simulink model "dynamics"  (R2024a)
settings: Solver=VariableStepAuto  StartTime=0.0  StopTime=10.0  RelTol=1e-3
values from neighbouring files (symbols this model uses):
  Arm = [ ... (first row only)    [launch.m]
  CDDrone = 0.01    [launch.m]
  CDval = 0.008    [launch.m]
  g = 9.81    [launch.m]
  m = 1    [launch.m]
  prop_inertia = (1/12) * 0.015 * 0.127^2    (= 2.016125e-05)    [launch.m]
  R = 0.127    [launch.m]
  rotorRPMMax = 10000    [launch.m]
  rotorTimeConst = 0.05    [launch.m]
  SampleTime = 0.004    [launch.m]
  tilt_speed = [0; pi/4; 0]    [launch.m]
undefined symbols (not defined in the file or in its folder): contact, control, ddx, ddy, ddz, dx, dy, dz, lastVh, p, pitch, q, r, roll, X, Y, yaw, Z
libraries: simulink x2, shared6dof x1, simulink_extras x1, sharedutil x1, matrix_library x1
settings Model: Creator=tommy  LastModifiedBy=tommy

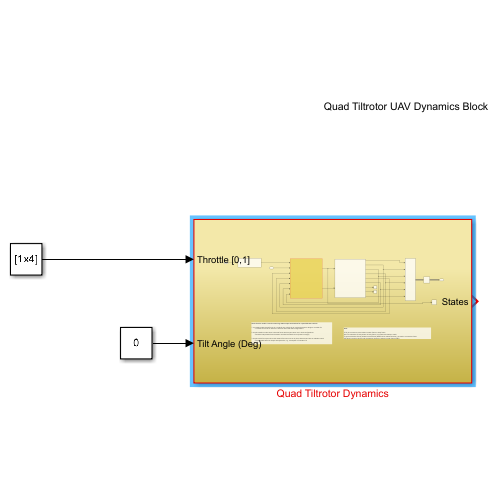
[thumbnail: Simulink's stored preview of the top-level diagram]
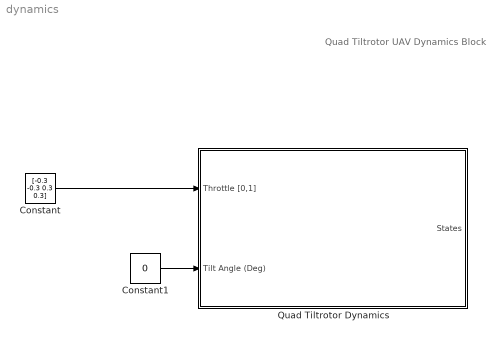
== system dynamics ==
  note: Quad Tiltrotor UAV Dynamics Block
  Constant : Constant  Value=[-0.3 -0.3 0.3 0.3]
  Constant1 : Constant  Value=0
  Quad Tiltrotor Dynamics : Subsystem
  wires:
  Constant/1 -> Quad Tiltrotor Dynamics/1(Throttle [0,1])
  Constant1/1 -> Quad Tiltrotor Dynamics/2(Tilt Angle (Deg))

== system dynamics/Quad Tiltrotor Dynamics ==
  note: Goals for this model : A novel vortex ring state escape mechanism for a quad tilt-rotor vehicle.
      |
      | 1. accurately portray thrust forces in a quad-tilt rotor vehicle in an in-place descent to design a controller for
      | - curve fits from CFD for descent in both non tilted and tilted configurations
      |
      | 2. simple transition model since horizontal forces and torques cancel out in both configurations
      | - transition interpolates forces between non tilted and tilted curves (based on angle)
      |
      | 3. simple model for torques since this research focuses more on in-place descents and less on attitude control
      | - torque model based on simple aerodynamics, e.g., assumption of constant Cd
  note: Note:
      |
      | DCM_be converts a vector written in earth frame to body frame
      | Abe is acceleration of body written in body frame, but measured relative to earth.
      | To get acceleration of body written in earth frame (NED fixed on takeoff location), we need to convert the frame.
      | IMU block's angular velocity and acceleration inputs are written in earth frame (NED)
  Throttle [0,1] : Inport
  Tilt Angle (Deg) : Inport  Port=2
  6DOF (Quaternion) : shared6dof/6DOF (Euler Angles)  units=Metric (MKS)  mtype=Fixed  rep=Quaternion  xme_0=init.posNED  Vm_0=init.vb  eul_0=init.euler  pm_0=init.angRates  mass_0=m  mass_e=0.5  mass_f=2.0  inertia=inertia  inertia_e=eye(3)  inertia_f=2*eye(3)  k_quat=1  vre_flag=on  abi_flag=on  aMode=0  xme_statename=''  Vm_statename=''  eul_statename=''  quat_statename=''  pm_statename=''  mass_statename=''
      settings: LibrarySourceBlock=aerolib6dof2/6DOF (Quaternion)
  Airframe : Subsystem
      mask Display: image('PX4-Quad-X-Motor-Configuration-33.png', [5,0,0,0,80,50]);
  Motor Model : Subsystem
  Rate Transition : RateTransition  OutPortSampleTime=SampleTime
  Scope : Scope
  States Bus : Subsystem
  Terminator : Terminator
  Terminator1 : Terminator
  States : Outport
  wires:
  States Bus/1(States) -> Rate Transition/1
  Rate Transition/1 -> States/1
  6DOF (Quaternion)/7 -> Terminator/1
  6DOF (Quaternion)/4 -> Airframe/4(DCMbe), States Bus/4(DCMbe)
  6DOF (Quaternion)/6 -> Airframe/6(Wb), States Bus/5(Wb)
  Airframe/1(F_cg) -> Scope/1, 6DOF (Quaternion)/1
  6DOF (Quaternion)/2 -> Airframe/5(Xe), States Bus/2(Xe)
  Airframe/2(M_cg) -> 6DOF (Quaternion)/2
  6DOF (Quaternion)/9 -> States Bus/6(acc_lnav)
  6DOF (Quaternion)/5 -> Airframe/3(Vb)
  6DOF (Quaternion)/8 -> Terminator1/1
  6DOF (Quaternion)/3 -> Airframe/7(rpy), States Bus/3(rpy)
  6DOF (Quaternion)/1 -> States Bus/1(Ve)
  Tilt Angle (Deg)/1 -> Airframe/2(Tilt Angle (Deg))
  Throttle [0,1]/1 -> Motor Model/1(Throttle)
  Motor Model/1(RPM) -> Airframe/1(rpm)

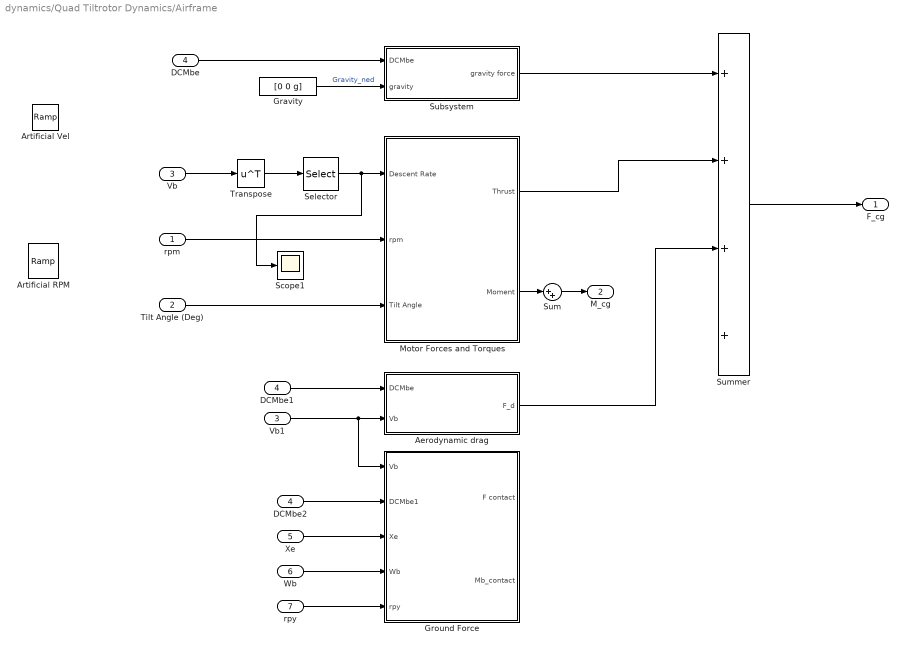
== system dynamics/Quad Tiltrotor Dynamics/Airframe ==
  rpm : Inport
  Tilt Angle (Deg) : Inport  Port=2
  Vb : Inport  Port=3
  DCMbe : Inport  Port=4
  Xe : Inport  Port=5
  Wb : Inport  Port=6
  rpy : Inport  Port=7
  Aerodynamic drag : Subsystem
  Artificial RPM : simulink/Sources/Ramp  slope=[0;-0;0;-0]  start=0  InitialOutput=[-3000; 3000; -2000; 2000]  VectorParams1D=off
  Artificial Vel : simulink/Sources/Ramp  slope=[0;0;0]  start=0  InitialOutput=[0;0;0]  VectorParams1D=off
  DCMbe1 : InportShadow  Port=4
  DCMbe2 : InportShadow  Port=4
  Gravity : Constant  Value=[0 0 g]
  Ground Force : Subsystem
  Motor Forces and Torques : Subsystem
  Scope1 : Scope
  Selector : Selector  InputPortWidth=3  IndexOptions=Index vector (dialog)  Indices=[3]  OutputSizes=1
  Subsystem : Subsystem
  Sum : Sum  Inputs=|++
  Summer : Sum  Inputs=++++
  Transpose : Math  Operator=transpose
  Vb1 : InportShadow  Port=3
  F_cg : Outport
  M_cg : Outport  Port=2
  wires:
  Subsystem/1(gravity force) -> Summer/1
  rpm/1 -> Motor Forces and Torques/2(rpm)
  Gravity/1 -> Subsystem/2(gravity)  "Gravity_ned"
  DCMbe/1 -> Subsystem/1(DCMbe)
  Transpose/1 -> Selector/1
  Selector/1 -> Scope1/1, Motor Forces and Torques/1(Descent Rate)
  Tilt Angle (Deg)/1 -> Motor Forces and Torques/3(Tilt Angle)
  Summer/1 -> F_cg/1
  Vb/1 -> Transpose/1
  DCMbe2/1 -> Ground Force/2(DCMbe1)
  Vb1/1 -> Ground Force/1(Vb), Aerodynamic drag/2(Vb)
  Xe/1 -> Ground Force/3(Xe)
  Aerodynamic drag/1(F_d) -> Summer/3
  Sum/1 -> M_cg/1
  rpy/1 -> Ground Force/5(rpy)
  Wb/1 -> Ground Force/4(Wb)
  DCMbe1/1 -> Aerodynamic drag/1(DCMbe)
  Motor Forces and Torques/2(Moment) -> Sum/1
  Motor Forces and Torques/1(Thrust) -> Summer/2

== system dynamics/Quad Tiltrotor Dynamics/Motor Model ==
  Throttle : Inport
  Demux : Demux
  Gain : Gain  Gain=[-1;-1;1;1]
  Mux : Mux
  Transfer Fcn{,2..4} (4 alike) : TransferFcn  Numerator=[rotorRPMMax]  Denominator=[rotorTimeConst 1]
  RPM : Outport
  wires:
  Mux/1 -> Gain/1
  Transfer Fcn/1 -> Mux/4
  Demux/4 -> Transfer Fcn/1
  Transfer Fcn3/1 -> Mux/2
  Transfer Fcn2/1 -> Mux/3
  Demux/1 -> Transfer Fcn4/1
  Demux/3 -> Transfer Fcn2/1
  Demux/2 -> Transfer Fcn3/1
  Transfer Fcn4/1 -> Mux/1
  Gain/1 -> RPM/1
  Throttle/1 -> Demux/1

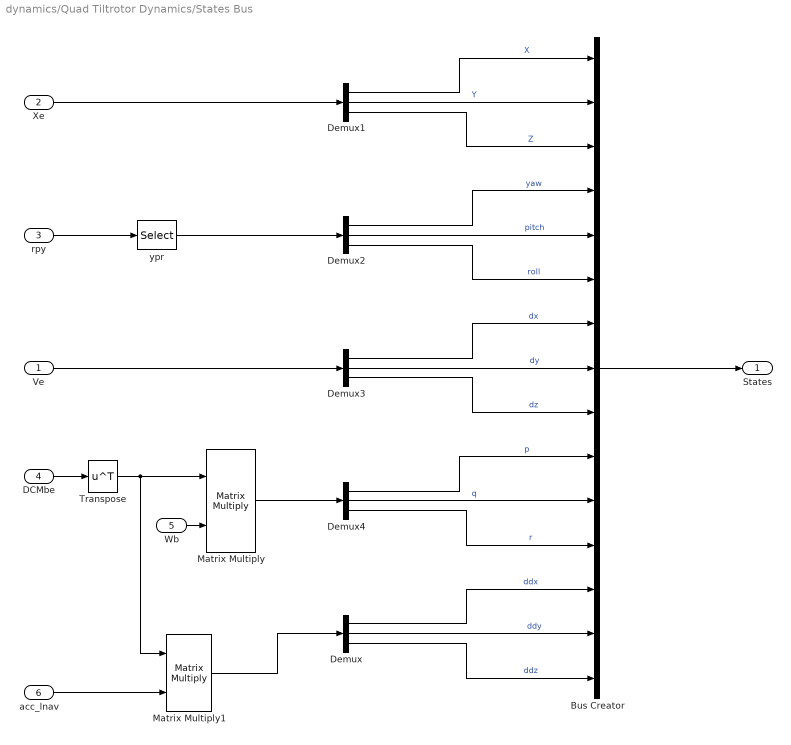
== system dynamics/Quad Tiltrotor Dynamics/States Bus ==
  Ve : Inport
  Xe : Inport  Port=2
  rpy : Inport  Port=3
  DCMbe : Inport  Port=4
  Wb : Inport  Port=5
  acc_lnav : Inport  Port=6
  Bus Creator : BusCreator  Inputs=X,Y,Z,yaw,pitch,roll,dx,dy,dz,p,q,r,ddx,ddy,ddz
  Demux{,1..4} (5 alike) : Demux  Outputs=3
  Matrix Multiply : Product  Multiplication=Matrix(*)
  Matrix Multiply1 : Product  Multiplication=Matrix(*)
  Transpose : Math  Operator=transpose
  ypr : Selector  InputPortWidth=3  IndexOptions=Index vector (dialog)  Indices=[3 2 1]  OutputSizes=1
  States : Outport
  wires:
  Demux1/1 -> Bus Creator/1  "X"
  Demux1/2 -> Bus Creator/2  "Y"
  rpy/1 -> ypr/1
  Demux2/2 -> Bus Creator/5  "pitch"
  Demux3/2 -> Bus Creator/8  "dy"
  Demux2/3 -> Bus Creator/6  "roll"
  Ve/1 -> Demux3/1
  Demux2/1 -> Bus Creator/4  "yaw"
  Demux1/3 -> Bus Creator/3  "Z"
  Demux3/1 -> Bus Creator/7  "dx"
  Demux4/2 -> Bus Creator/11  "q"
  Demux3/3 -> Bus Creator/9  "dz"
  Demux4/3 -> Bus Creator/12  "r"
  Demux4/1 -> Bus Creator/10  "p"
  Bus Creator/1 -> States/1
  Xe/1 -> Demux1/1
  Demux/3 -> Bus Creator/15  "ddz"
  Demux/2 -> Bus Creator/14  "ddy"
  Demux/1 -> Bus Creator/13  "ddx"
  Matrix Multiply/1 -> Demux4/1
  DCMbe/1 -> Transpose/1
  Transpose/1 -> Matrix Multiply1/1, Matrix Multiply/1
  Wb/1 -> Matrix Multiply/2
  acc_lnav/1 -> Matrix Multiply1/2
  Matrix Multiply1/1 -> Demux/1
  ypr/1 -> Demux2/1

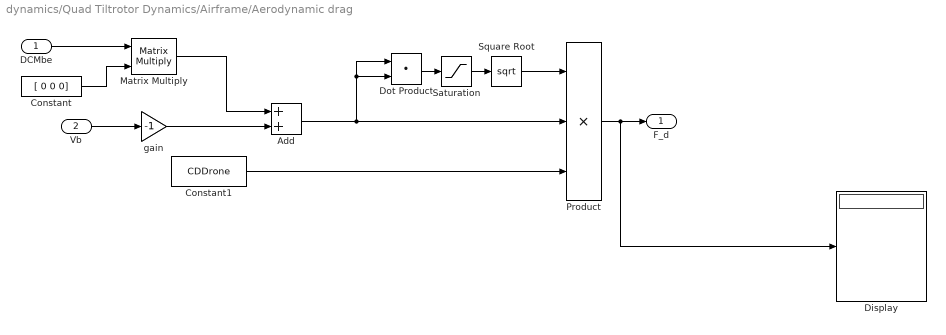
== system dynamics/Quad Tiltrotor Dynamics/Airframe/Aerodynamic drag ==
  DCMbe : Inport
  Vb : Inport  Port=2
  Add : Sum
  Constant : Constant  Value=[ 0 0 0]
  Constant1 : Constant  Value=CDDrone
  Display : Display
  Dot Product : DotProduct  OutDataTypeStr=Inherit: Inherit via internal rule
  Matrix Multiply : Product  Multiplication=Matrix(*)
  Product : Product  Inputs=3
  Saturation : Saturate  UpperLimit=inf  LowerLimit=0.0001
  Square Root : Sqrt
  gain : Gain  Gain=-1
  F_d : Outport
  wires:
  Saturation/1 -> Square Root/1
  Vb/1 -> gain/1
  Dot Product/1 -> Saturation/1
  Square Root/1 -> Product/1
  Constant1/1 -> Product/3
  DCMbe/1 -> Matrix Multiply/1
  Constant/1 -> Matrix Multiply/2
  gain/1 -> Add/2
  Matrix Multiply/1 -> Add/1
  Add/1 -> Dot Product/1, Dot Product/2, Product/2
  Product/1 -> Display/1, F_d/1

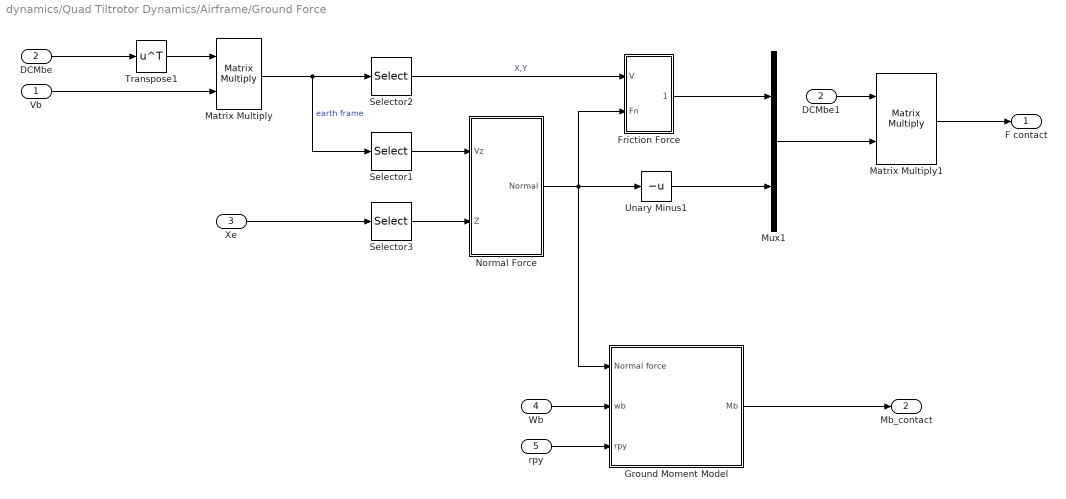
== system dynamics/Quad Tiltrotor Dynamics/Airframe/Ground Force ==
  Vb : Inport
  DCMbe1 : Inport  Port=2
  Xe : Inport  Port=3
  Wb : Inport  Port=4
  rpy : Inport  Port=5
  DCMbe : InportShadow  Port=2
  Friction Force : Subsystem
  Ground Moment Model : Subsystem
  Matrix Multiply : Product  Multiplication=Matrix(*)
  Matrix Multiply1 : Product  Multiplication=Matrix(*)
  Mux1 : Mux  Inputs=2
  Normal Force : Subsystem
  Selector1 : Selector  InputPortWidth=3  IndexOptions=Index vector (dialog)  Indices=[3]  OutputSizes=1
  Selector2 : Selector  InputPortWidth=3  IndexOptions=Index vector (dialog)  Indices=[1,2]  OutputSizes=1
  Selector3 : Selector  InputPortWidth=3  IndexOptions=Index vector (dialog)  Indices=[3]  OutputSizes=1
  Transpose1 : Math  Operator=transpose
  Unary Minus1 : UnaryMinus
  F contact : Outport
  Mb_contact : Outport  Port=2
  wires:
  Matrix Multiply1/1 -> F contact/1
  Friction Force/1(Friction) -> Mux1/1
  Xe/1 -> Selector3/1
  Vb/1 -> Matrix Multiply/2
  Selector3/1 -> Normal Force/2(Z)
  Matrix Multiply/1 -> Selector1/1, Selector2/1  "earth frame"
  Mux1/1 -> Matrix Multiply1/2
  Selector2/1 -> Friction Force/1(V)  "X,Y"
  Selector1/1 -> Normal Force/1(Vz)
  DCMbe1/1 -> Matrix Multiply1/1
  DCMbe/1 -> Transpose1/1
  Transpose1/1 -> Matrix Multiply/1
  Unary Minus1/1 -> Mux1/2
  Normal Force/1(Normal) -> Ground Moment Model/1(Normal force), Unary Minus1/1, Friction Force/2(Fn)
  Wb/1 -> Ground Moment Model/2(wb)
  rpy/1 -> Ground Moment Model/3(rpy)
  Ground Moment Model/1(Mb) -> Mb_contact/1

== system dynamics/Quad Tiltrotor Dynamics/Airframe/Motor Forces and Torques ==
  Descent Rate : Inport
  rpm : Inport  Port=2
  Tilt Angle : Inport  Port=3
  Constant1 : Constant  Value=Arm
  Degrees to Radians : simulink_extras/Transformations/Degrees to Radians
  Multirotor Subsystem : Subsystem  TreatAsAtomicUnit=on
  Sum of Elements : Sum  Inputs=+  CollapseMode=Specified dimension  CollapseDim=2
  Sum of Elements1 : Sum  Inputs=+  CollapseMode=Specified dimension  CollapseDim=2
  rho : Constant  Value=1.225
  Thrust : Outport
  Moment : Outport  Port=2
  wires:
  Tilt Angle/1 -> Degrees to Radians/1
  Constant1/1 -> Multirotor Subsystem/4(Arm)
  Degrees to Radians/1 -> Multirotor Subsystem/5(Tilt Angle (rad))
  Sum of Elements/1 -> Thrust/1
  Sum of Elements1/1 -> Moment/1
  Descent Rate/1 -> Multirotor Subsystem/1(Descent Rate (+ve down))
  rho/1 -> Multirotor Subsystem/2(rho)
  Multirotor Subsystem/2(Moment) -> Sum of Elements1/1
  Multirotor Subsystem/1(Thrust) -> Sum of Elements/1
  rpm/1 -> Multirotor Subsystem/3(rpm)

== system dynamics/Quad Tiltrotor Dynamics/Airframe/Subsystem ==
  DCMbe : Inport
  gravity : Inport  Port=2  Unit=m/s^2
  Gain1 : Gain  Gain=m
  Product : Product  Multiplication=Matrix(*)
  gravity force : Outport  Unit=N  VectorParamsAs1DForOutWhenUnconnected=off
  wires:
  gravity/1 -> Gain1/1
  Product/1 -> gravity force/1
  DCMbe/1 -> Product/1
  Gain1/1 -> Product/2  "gravity force NED"

== system dynamics/Quad Tiltrotor Dynamics/Airframe/Ground Force/Friction Force ==
  V : Inport
  Fn : Inport  Port=2
  Product : Product
  Saturation : Saturate  UpperLimit=contact.translation.maxFriction  LowerLimit=-contact.translation.maxFriction
  Soft Coulomb Friction : Subsystem
  Unary Minus : UnaryMinus
  Friction : Outport
  wires:
  Fn/1 -> Product/2
  Soft Coulomb Friction/1(Out1) -> Product/1
  Product/1 -> Unary Minus/1
  V/1 -> Soft Coulomb Friction/1(In1)
  Unary Minus/1 -> Saturation/1
  Saturation/1 -> Friction/1

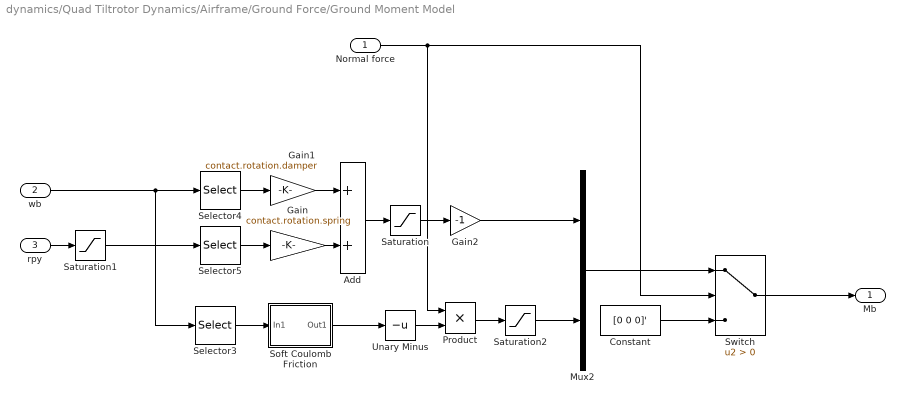
== system dynamics/Quad Tiltrotor Dynamics/Airframe/Ground Force/Ground Moment Model ==
  Normal force : Inport
  wb : Inport  Port=2
  rpy : Inport  Port=3
  Add : Sum
  Constant : Constant  Value=[0 0 0]'
  Gain : Gain  Gain=contact.rotation.spring
  Gain1 : Gain  Gain=contact.rotation.damper
  Gain2 : Gain  Gain=-1
  Mux2 : Mux  Inputs=2
  Product : Product
  Saturation : Saturate  UpperLimit=control.rotation.maxMoment  LowerLimit=-control.rotation.maxMoment
  Saturation1 : Saturate  UpperLimit=20*pi/180  LowerLimit=-20*pi/180
  Saturation2 : Saturate  UpperLimit=control.rotation.maxMoment  LowerLimit=-control.rotation.maxMoment
  Selector3 : Selector  InputPortWidth=3  IndexOptions=Index vector (dialog)  Indices=[3]  OutputSizes=1
  Selector4 : Selector  InputPortWidth=3  IndexOptions=Index vector (dialog)  Indices=[1, 2]  OutputSizes=1
  Selector5 : Selector  InputPortWidth=3  IndexOptions=Index vector (dialog)  Indices=[1, 2]  OutputSizes=1
  Soft Coulomb Friction : Subsystem
  Switch : Switch  Criteria=u2 > Threshold  SaturateOnIntegerOverflow=off  InputSameDT=off
  Unary Minus : UnaryMinus
  Mb : Outport
  wires:
  Gain2/1 -> Mux2/1
  Add/1 -> Saturation/1
  Gain/1 -> Add/2
  Saturation/1 -> Gain2/1
  Selector4/1 -> Gain1/1
  Gain1/1 -> Add/1
  Constant/1 -> Switch/3
  Selector5/1 -> Gain/1
  Switch/1 -> Mb/1
  Mux2/1 -> Switch/1
  Normal force/1 -> Product/1, Switch/2
  rpy/1 -> Saturation1/1
  Saturation1/1 -> Selector5/1
  wb/1 -> Selector4/1, Selector3/1
  Selector3/1 -> Soft Coulomb Friction/1(In1)
  Soft Coulomb Friction/1(Out1) -> Unary Minus/1
  Unary Minus/1 -> Product/2
  Product/1 -> Saturation2/1
  Saturation2/1 -> Mux2/2

== system dynamics/Quad Tiltrotor Dynamics/Airframe/Ground Force/Normal Force ==
  Vz : Inport
  Z : Inport  Port=2
  Add : Sum
  Constant : Constant  Value=0
  Damper Kp : Gain  Gain=-contact.translation.damper
  Saturation : Saturate  UpperLimit=contact.translation.maxNormal  LowerLimit=0
  Spring Kp : Gain  Gain=-contact.translation.spring
  Switch : Switch  Criteria=u2 > Threshold  SaturateOnIntegerOverflow=off  InputSameDT=off
  Unary Minus : UnaryMinus
  Unary Minus1 : UnaryMinus
  Normal : Outport
  wires:
  Constant/1 -> Switch/1
  Z/1 -> Unary Minus/1
  Switch/1 -> Saturation/1
  Damper Kp/1 -> Add/2
  Add/1 -> Switch/3
  Spring Kp/1 -> Add/1
  Vz/1 -> Unary Minus1/1
  Saturation/1 -> Normal/1
  Unary Minus/1 -> Spring Kp/1, Switch/2
  Unary Minus1/1 -> Damper Kp/1

== system dynamics/Quad Tiltrotor Dynamics/Airframe/Motor Forces and Torques/Multirotor Subsystem ==
  Descent Rate (+ve down) : Inport
  rho : Inport  Port=2
  rpm : Inport  Port=3  Partition=on  PartitionDimension=1  PartitionWidth=1  PartitionOffset=0
  Arm : Inport  Port=4  Partition=on  PartitionDimension=2  PartitionWidth=1  PartitionOffset=0
  Tilt Angle (rad) : Inport  Port=5
  For Each : ForEach  DisableCoverage=on
  Rotor Subsystem : Subsystem
  Thrust : Outport  ConcatenationDimension=2
  Moment : Outport  Port=2  ConcatenationDimension=2
  wires:
  Rotor Subsystem/4(Mxyz) -> Moment/1  "Moment"
  Arm/1 -> Rotor Subsystem/4(Arm)
  Descent Rate (+ve down)/1 -> Rotor Subsystem/1(Descent Rate (+ve down))
  rho/1 -> Rotor Subsystem/2(rho)
  Rotor Subsystem/3(Fxyz) -> Thrust/1  "Thrust"
  rpm/1 -> Rotor Subsystem/3(rpm)
  Tilt Angle (rad)/1 -> Rotor Subsystem/5(Tilt Angle (rad))

== system dynamics/Quad Tiltrotor Dynamics/Airframe/Ground Force/Friction Force/Soft Coulomb Friction ==
  note: Pennestrì, E., Rossi, V., Salvini, P. et al. Review and comparison of dry friction force models. Nonlinear Dyn 83, 1785–1801 (2016). https://doi.org/10.1007/s11071-015-2485-3
  In1 : Inport
  Tanh : Trigonometry  Operator=tanh
  friction coefficient : Gain  Gain=contact.translation.friction
  vd : Gain  Gain=1/contact.translation.vd
  Out1 : Outport
  wires:
  In1/1 -> vd/1
  vd/1 -> Tanh/1
  Tanh/1 -> friction coefficient/1
  friction coefficient/1 -> Out1/1

== system dynamics/Quad Tiltrotor Dynamics/Airframe/Ground Force/Ground Moment Model/Soft Coulomb Friction ==
  note: Pennestrì, E., Rossi, V., Salvini, P. et al. Review and comparison of dry friction force models. Nonlinear Dyn 83, 1785–1801 (2016). https://doi.org/10.1007/s11071-015-2485-3
  In1 : Inport
  Tanh : Trigonometry  Operator=tanh
  friction coefficient : Gain  Gain=control.rotation.friction
  vd : Gain  Gain=1/control.rotation.vd
  Out1 : Outport
  wires:
  In1/1 -> vd/1
  vd/1 -> Tanh/1
  Tanh/1 -> friction coefficient/1
  friction coefficient/1 -> Out1/1

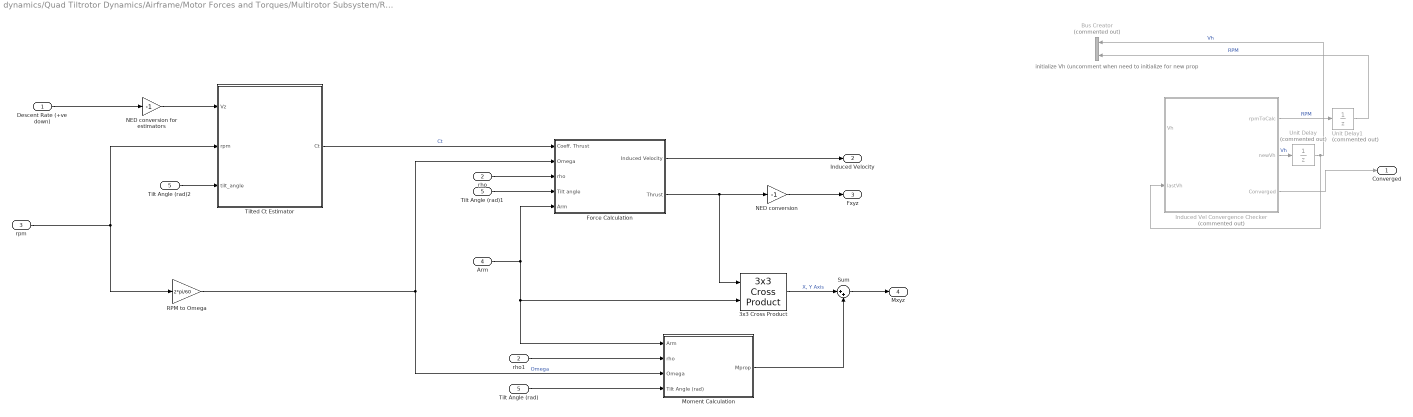
== system dynamics/Quad Tiltrotor Dynamics/Airframe/Motor Forces and Torques/Multirotor Subsystem/Rotor Subsystem ==
  note: initialize Vh (uncomment when need to initialize for new prop
  Descent Rate (+ve down) : Inport
  rho : Inport  Port=2
  rpm : Inport  Port=3
  Arm : Inport  Port=4
  Tilt Angle (rad) : Inport  Port=5
  3x3 Cross Product : sharedutil/3x3 Cross Product  aMode=aMode
      settings: LibrarySourceBlock=aerolibutil/3x3 Cross Product
  Bus Creator : BusCreator  Commented=on  Inputs=2
  Force Calculation : Subsystem
  Induced Vel Convergence Checker : MATLAB Function  Commented=on  TreatAsAtomicUnit=on  mask{VhInit=4.7, ConvThresh=1e-4}
      mask prompts: VhInit "Initial Vh Guess"; ConvThresh "Convergence Threshold"
  Moment Calculation : Subsystem
  NED conversion : Gain  Gain=-1
  NED conversion for estimators : Gain  Gain=-1
  RPM to Omega : Gain  Gain=2*pi/60
  Sum : Sum  Inputs=|++
  Tilt Angle (rad)1 : InportShadow  Port=5
  Tilt Angle (rad)2 : InportShadow  Port=5
  Tilted Ct Estimator : Subsystem
  Unit Delay : UnitDelay  Commented=on  InitialCondition=lastVh  SampleTime=0.001  HasFrameUpgradeWarning=on
  Unit Delay1 : UnitDelay  Commented=on  InitialCondition=1  SampleTime=0.001  HasFrameUpgradeWarning=on
  rho1 : InportShadow  Port=2
  Converged : Outport
  Induced Velocity : Outport  Port=2
  Fxyz : Outport  Port=3
  Mxyz : Outport  Port=4
  wires:
  Tilted Ct Estimator/1(Ct) -> Force Calculation/1(Coeff. Thrust)  "Ct"
  Unit Delay/1 -> Bus Creator/1, Induced Vel Convergence Checker/2(lastVh)  "Vh"
  Induced Vel Convergence Checker/3(Converged) -> Converged/1
  RPM to Omega/1 -> Moment Calculation/3(Omega), Force Calculation/2(Omega)  "Omega"
  rho/1 -> Force Calculation/3(rho)
  Induced Vel Convergence Checker/2(newVh) -> Unit Delay/1  "Vh"
  rpm/1 -> RPM to Omega/1, Tilted Ct Estimator/2(rpm)
  Descent Rate (+ve down)/1 -> NED conversion for estimators/1
  Unit Delay1/1 -> Bus Creator/2  "RPM"
  Induced Vel Convergence Checker/1(rpmToCalc) -> Unit Delay1/1  "RPM"
  Force Calculation/1(Induced Velocity) -> Induced Velocity/1
  Force Calculation/2(Thrust) -> NED conversion/1, 3x3 Cross Product/1
  3x3 Cross Product/1 -> Sum/1  "X, Y Axis"
  rho1/1 -> Moment Calculation/2(rho)
  Arm/1 -> 3x3 Cross Product/2, Moment Calculation/1(Arm), Force Calculation/5(Arm)
  Moment Calculation/1(Mprop) -> Sum/2
  Sum/1 -> Mxyz/1
  NED conversion/1 -> Fxyz/1
  Tilt Angle (rad)/1 -> Moment Calculation/4(Tilt Angle (rad))
  Tilt Angle (rad)1/1 -> Force Calculation/4(Tilt angle)
  NED conversion for estimators/1 -> Tilted Ct Estimator/1(Vz)
  Tilt Angle (rad)2/1 -> Tilted Ct Estimator/3(tilt_angle)

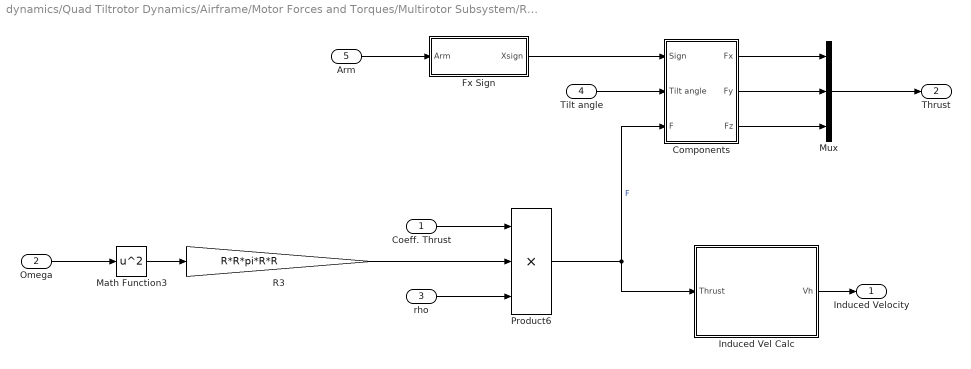
== system dynamics/Quad Tiltrotor Dynamics/Airframe/Motor Forces and Torques/Multirotor Subsystem/Rotor Subsystem/Force Calculation ==
  Coeff. Thrust : Inport
  Omega : Inport  Port=2
  rho : Inport  Port=3
  Tilt angle : Inport  Port=4
  Arm : Inport  Port=5
  Components : Subsystem
  Fx Sign : Subsystem
  Induced Vel Calc : Subsystem
  Math Function3 : Math  Operator=square  SignedPower=on
  Mux : Mux  Inputs=3
  Product6 : Product  Inputs=3
  R3 : Gain  Gain=R*R*pi*R*R
  Induced Velocity : Outport
  Thrust : Outport  Port=2
  wires:
  Coeff. Thrust/1 -> Product6/1
  Math Function3/1 -> R3/1
  Induced Vel Calc/1(Vh) -> Induced Velocity/1
  R3/1 -> Product6/2
  rho/1 -> Product6/3
  Omega/1 -> Math Function3/1
  Product6/1 -> Components/3(F), Induced Vel Calc/1(Thrust)  "F"
  Arm/1 -> Fx Sign/1(Arm)
  Mux/1 -> Thrust/1
  Fx Sign/1(Xsign) -> Components/1(Sign)
  Tilt angle/1 -> Components/2(Tilt angle)
  Components/1(Fx) -> Mux/1
  Components/2(Fy) -> Mux/2
  Components/3(Fz) -> Mux/3

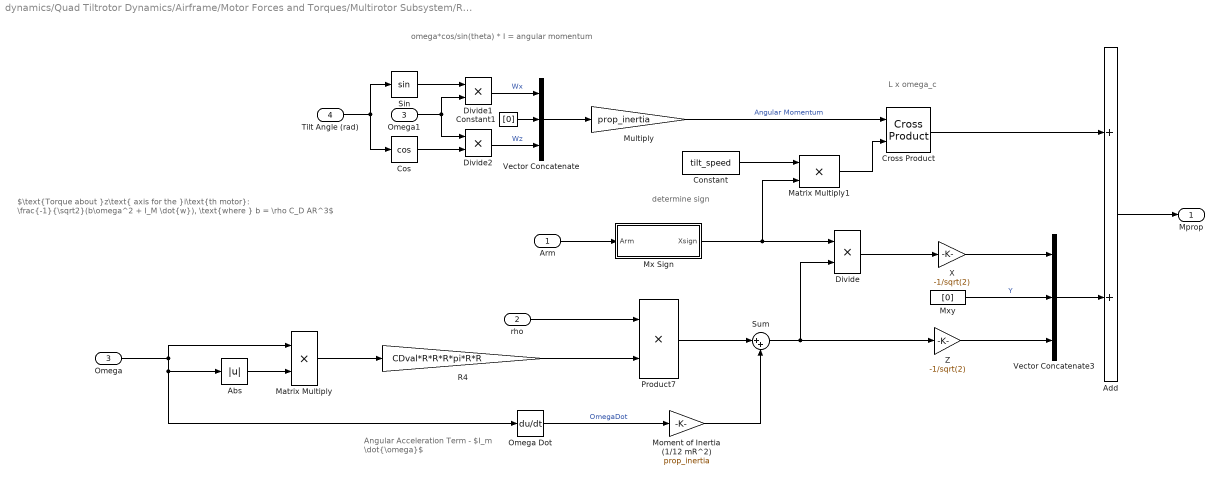
== system dynamics/Quad Tiltrotor Dynamics/Airframe/Motor Forces and Torques/Multirotor Subsystem/Rotor Subsystem/Moment Calculation ==
  note: determine sign
  note: L x omega_c
  note: omega*cos/sin(theta) * I = angular momentum
  note: $\text{Torque about }z\text{ axis for the }i\text{th motor}: \frac{-1}{\sqrt2}(b\omega^2 + I_M \dot{w}), \text{where } b = \rho C_D AR^3$
  note: Angular Acceleration Term - $I_m \dot{\omega}$
  Arm : Inport
  rho : Inport  Port=2
  Omega : Inport  Port=3
  Tilt Angle (rad) : Inport  Port=4
  Abs : Abs  SaturateOnIntegerOverflow=off
  Add : Sum
  Constant : Constant  Value=tilt_speed
  Constant1 : Constant  Value=[0]
  Cos : Trigonometry  Operator=cos
  Cross Product : matrix_library/Cross Product
  Divide : Product  Inputs=**
  Divide1 : Product  Inputs=**
  Divide2 : Product  Inputs=**
  Matrix Multiply : Product
  Matrix Multiply1 : Product
  Moment of Inertia (1/12 mR^2) : Gain  Gain=prop_inertia
  Multiply : Gain  Gain=prop_inertia
  Mx Sign : Subsystem
  Mxy : Constant  Value=[0]
  Omega Dot : Derivative
  Omega1 : InportShadow  Port=3
  Product7 : Product
  R4 : Gain  Gain=CDval*R*R*R*pi*R*R
  Sin : Trigonometry
  Sum : Sum  Inputs=|++
  Vector Concatenate : Concatenate  NumInputs=3
  Vector Concatenate3 : Concatenate  NumInputs=3
  X : Gain  Gain=-1/sqrt(2)
  Z : Gain  Gain=-1/sqrt(2)
  Mprop : Outport
  wires:
  R4/1 -> Product7/2
  rho/1 -> Product7/1
  Omega/1 -> Omega Dot/1, Abs/1, Matrix Multiply/1
  Omega Dot/1 -> Moment of Inertia (1/12 mR^2)/1  "OmegaDot"
  Sum/1 -> Z/1, Divide/2
  Product7/1 -> Sum/1
  Moment of Inertia (1/12 mR^2)/1 -> Sum/2
  Z/1 -> Vector Concatenate3/3
  Divide/1 -> X/1
  Mxy/1 -> Vector Concatenate3/2  "Y"
  Arm/1 -> Mx Sign/1(Arm)
  Mx Sign/1(Xsign) -> Divide/1, Matrix Multiply1/2
  Matrix Multiply/1 -> R4/1
  Abs/1 -> Matrix Multiply/2
  Tilt Angle (rad)/1 -> Cos/1, Sin/1
  Cos/1 -> Divide2/2
  Sin/1 -> Divide1/1
  Divide1/1 -> Vector Concatenate/1  "Wx"
  Vector Concatenate/1 -> Multiply/1
  Multiply/1 -> Cross Product/1  "Angular Momentum"
  Cross Product/1 -> Add/1
  Divide2/1 -> Vector Concatenate/3  "Wz"
  Constant1/1 -> Vector Concatenate/2
  Omega1/1 -> Divide2/1, Divide1/2
  Matrix Multiply1/1 -> Cross Product/2
  Constant/1 -> Matrix Multiply1/1
  X/1 -> Vector Concatenate3/1
  Vector Concatenate3/1 -> Add/2
  Add/1 -> Mprop/1

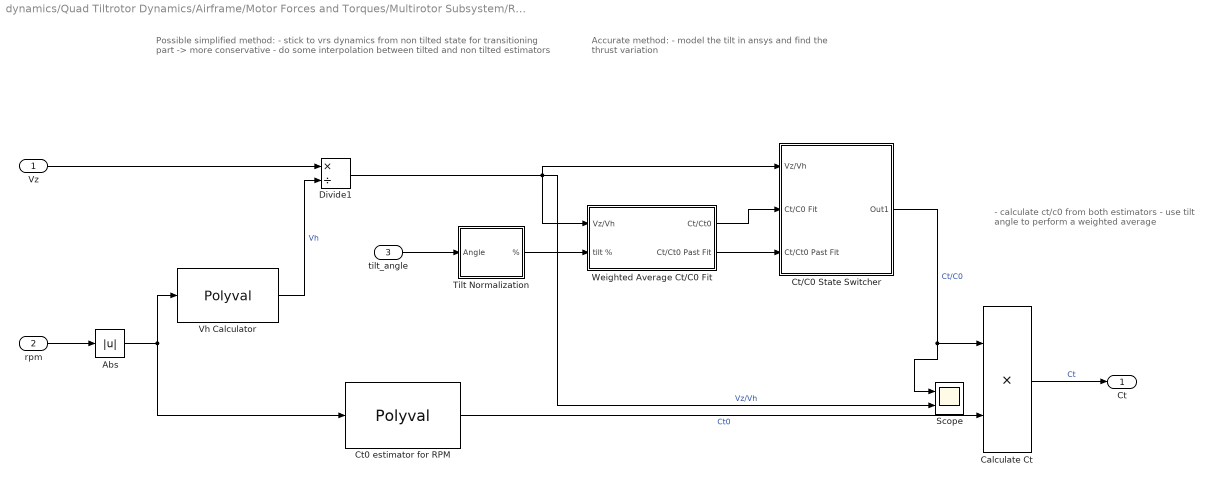
== system dynamics/Quad Tiltrotor Dynamics/Airframe/Motor Forces and Torques/Multirotor Subsystem/Rotor Subsystem/Tilted Ct Estimator ==
  note: - calculate ct/c0 from both estimators
      | - use tilt angle to perform a weighted average
  note: Accurate method:
      |
      | - model the tilt in ansys and find the thrust variation
  note: Possible simplified method:
      |
      | - stick to vrs dynamics from non tilted state for transitioning part -> more conservative
      | - do some interpolation between tilted and non tilted estimators
  Vz : Inport
  rpm : Inport  Port=2
  tilt_angle : Inport  Port=3
  Abs : Abs  SaturateOnIntegerOverflow=off
  Calculate Ct : Product  Inputs=**
  Ct/C0 State Switcher : Subsystem
  Ct0 estimator for RPM : Polyval  Coefs=[0.000000000012185, -0.000000274732884, 0.008305365728125]
  Divide1 : Product  Inputs=*/
  Scope : Scope  NumInputPorts=2
  Tilt Normalization : Subsystem
  Vh Calculator : Polyval  Coefs=[-5.17622414362771e-09, 0.000822973507549008, 0.0232660553338375]
  Weighted Average Ct/C0 Fit : Subsystem
  Ct : Outport
  wires:
  Vh Calculator/1 -> Divide1/2  "Vh"
  Ct/C0 State Switcher/1(Out1) -> Scope/1, Calculate Ct/1  "Ct/C0"
  Divide1/1 -> Scope/2, Ct/C0 State Switcher/1(" Vz/Vh"), Weighted Average Ct/C0 Fit/1(Vz/Vh)  "Vz/Vh"
  rpm/1 -> Abs/1
  Abs/1 -> Vh Calculator/1, Ct0 estimator for RPM/1
  Ct0 estimator for RPM/1 -> Calculate Ct/2  "Ct0"
  Vz/1 -> Divide1/1
  Calculate Ct/1 -> Ct/1  "Ct"
  Weighted Average Ct/C0 Fit/1(Ct/Ct0) -> Ct/C0 State Switcher/2(Ct/C0 Fit)
  tilt_angle/1 -> Tilt Normalization/1(Angle)
  Tilt Normalization/1(%) -> Weighted Average Ct/C0 Fit/2(tilt %)
  Weighted Average Ct/C0 Fit/2(Ct/Ct0 Past Fit) -> Ct/C0 State Switcher/3(Ct/Ct0 Past Fit)

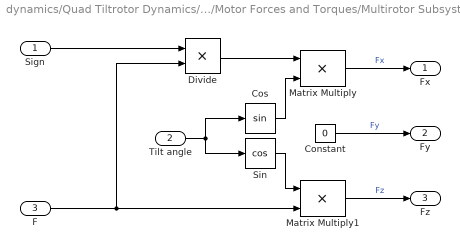
== system dynamics/Quad Tiltrotor Dynamics/Airframe/Motor Forces and Torques/Multirotor Subsystem/Rotor Subsystem/Force Calculation/Components ==
  Sign : Inport
  Tilt angle : Inport  Port=2
  F : Inport  Port=3
  Constant : Constant  Value=0
  Cos : Trigonometry
  Divide : Product  Inputs=**
  Matrix Multiply : Product
  Matrix Multiply1 : Product
  Sin : Trigonometry  Operator=cos
  Fx : Outport
  Fy : Outport  Port=2
  Fz : Outport  Port=3
  wires:
  Tilt angle/1 -> Cos/1, Sin/1
  Sign/1 -> Divide/1
  Sin/1 -> Matrix Multiply1/1
  Constant/1 -> Fy/1  "Fy"
  Cos/1 -> Matrix Multiply/2
  Matrix Multiply/1 -> Fx/1  "Fx"
  Divide/1 -> Matrix Multiply/1
  F/1 -> Matrix Multiply1/2, Divide/2
  Matrix Multiply1/1 -> Fz/1  "Fz"

== system dynamics/Quad Tiltrotor Dynamics/Airframe/Motor Forces and Torques/Multirotor Subsystem/Rotor Subsystem/Force Calculation/Fx Sign ==
  Arm : Inport
  Sign : Signum
  X selector : Selector  InputPortWidth=3  IndexOptions=Index vector (dialog)  Indices=[1]  OutputSizes=1
  Xsign : Outport
  wires:
  Arm/1 -> X selector/1
  X selector/1 -> Sign/1
  Sign/1 -> Xsign/1

== system dynamics/Quad Tiltrotor Dynamics/Airframe/Motor Forces and Torques/Multirotor Subsystem/Rotor Subsystem/Force Calculation/Induced Vel Calc ==
  Thrust : Inport
  Denom : Constant  Value=2*1.225*pi*R^2
  Divide : Product  Inputs=*/
  Saturation : Saturate  UpperLimit=inf  LowerLimit=0.0001
  Sqrt : Sqrt  OutDataTypeStr=double
  Vh : Outport
  wires:
  Denom/1 -> Divide/2
  Divide/1 -> Saturation/1
  Sqrt/1 -> Vh/1
  Thrust/1 -> Divide/1
  Saturation/1 -> Sqrt/1

== system dynamics/Quad Tiltrotor Dynamics/Airframe/Motor Forces and Torques/Multirotor Subsystem/Rotor Subsystem/Moment Calculation/Mx Sign ==
  Arm : Inport
  Sign : Signum
  X selector : Selector  InputPortWidth=3  IndexOptions=Index vector (dialog)  Indices=[1]  OutputSizes=1
  Xsign : Outport
  wires:
  Arm/1 -> X selector/1
  X selector/1 -> Sign/1
  Sign/1 -> Xsign/1

== system dynamics/Quad Tiltrotor Dynamics/Airframe/Motor Forces and Torques/Multirotor Subsystem/Rotor Subsystem/Tilted Ct Estimator/Ct//C0 State Switcher ==
  " Vz/Vh" : Inport
  Ct/C0 Fit : Inport  Port=2
  Ct/Ct0 Past Fit : Inport  Port=3
  Constant : Constant  Value=1.00463796511
  If : If  IfExpression=u1 >= -2 & u1 <= 0  ElseIfExpressions=u1 < -2
  If Action Subsystem : Subsystem  TreatAsAtomicUnit=on
  If Action Subsystem1 : Subsystem  TreatAsAtomicUnit=on
  If Action Subsystem2 : Subsystem  TreatAsAtomicUnit=on
  Merge : Merge  Inputs=3
  Out1 : Outport
  wires:
  If Action Subsystem1/1(" ") -> Merge/2
  If Action Subsystem2/1(Out1) -> Merge/3
  If/3 -> If Action Subsystem2/Action  "climb"
  If/1 -> If Action Subsystem/Action  "descent"
  If Action Subsystem/1(Out1) -> Merge/1
  " Vz/Vh"/1 -> If/1
  If/2 -> If Action Subsystem1/Action  "past curve fit"
  Merge/1 -> Out1/1
  Ct/C0 Fit/1 -> If Action Subsystem/1(In1)
  Constant/1 -> If Action Subsystem2/1("  ")
  Ct/Ct0 Past Fit/1 -> If Action Subsystem1/1(Inport)

== system dynamics/Quad Tiltrotor Dynamics/Airframe/Motor Forces and Torques/Multirotor Subsystem/Rotor Subsystem/Tilted Ct Estimator/Tilt Normalization ==
  Angle : Inport
  Constant1 : Constant  Value=pi/4
  Divide2 : Product  Inputs=*/
  % : Outport
  wires:
  Constant1/1 -> Divide2/2
  Divide2/1 -> %/1
  Angle/1 -> Divide2/1

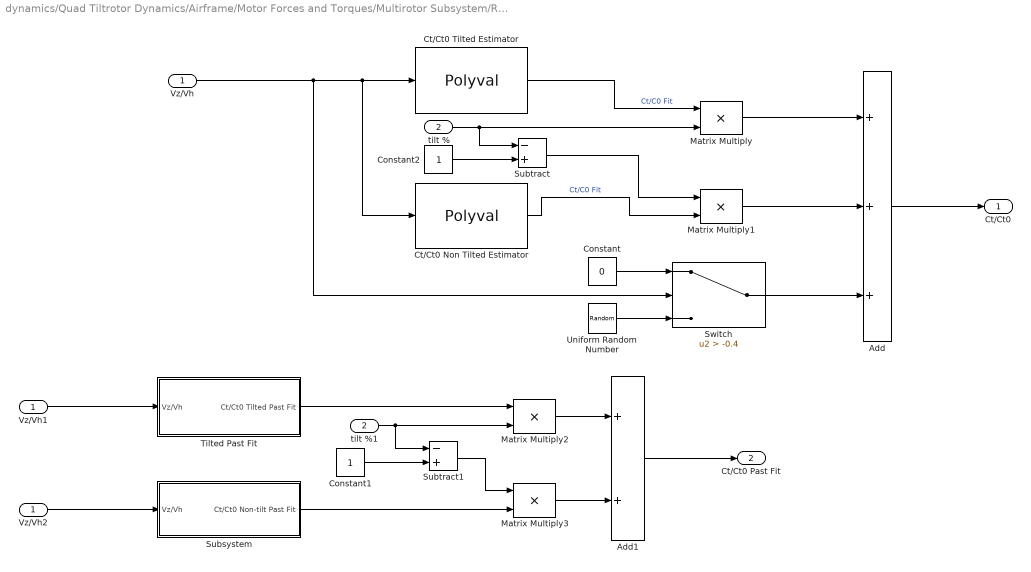
== system dynamics/Quad Tiltrotor Dynamics/Airframe/Motor Forces and Torques/Multirotor Subsystem/Rotor Subsystem/Tilted Ct Estimator/Weighted Average Ct//C0 Fit ==
  Vz/Vh : Inport
  tilt % : Inport  Port=2
  Add : Sum  Inputs=+++
  Add1 : Sum
  Constant : Constant  Value=0
  Constant1 : Constant
  Constant2 : Constant
  Ct/Ct0 Non Tilted Estimator : Polyval  Coefs=[0.147117704259973, 0.135195473604728, -0.341999514591595, -0.246799876690693, 0.999678014049876]
  Ct/Ct0 Tilted Estimator : Polyval  Coefs=[-0.012716815691322, -0.022830541813396, 0.156313447084851, -0.031641009616291, 1.004637965110952]
  Matrix Multiply{,1..3} (4 alike) : Product
  Subsystem : Subsystem
  Subtract : Sum  Inputs=-+
  Subtract1 : Sum  Inputs=-+
  Switch : Switch  Criteria=u2 > Threshold  Threshold=-0.4  SaturateOnIntegerOverflow=off  InputSameDT=off
  Tilted Past Fit : Subsystem
  Uniform Random Number : UniformRandomNumber  SampleTime=SampleTime
  Vz/Vh1 : InportShadow
  Vz/Vh2 : InportShadow
  tilt %1 : InportShadow  Port=2
  Ct/Ct0 : Outport
  Ct/Ct0 Past Fit : Outport  Port=2
  wires:
  Ct/Ct0 Tilted Estimator/1 -> Matrix Multiply/1  "Ct/C0 Fit"
  Vz/Vh/1 -> Switch/2, Ct/Ct0 Tilted Estimator/1, Ct/Ct0 Non Tilted Estimator/1
  Matrix Multiply/1 -> Add/1
  Ct/Ct0 Non Tilted Estimator/1 -> Matrix Multiply1/2  "Ct/C0 Fit"
  Matrix Multiply1/1 -> Add/2
  Subtract/1 -> Matrix Multiply1/1
  Add/1 -> Ct/Ct0/1
  Vz/Vh1/1 -> Tilted Past Fit/1(Vz/Vh)
  Vz/Vh2/1 -> Subsystem/1(" Vz/Vh")
  Add1/1 -> Ct/Ct0 Past Fit/1
  Constant2/1 -> Subtract/2
  tilt %/1 -> Subtract/1, Matrix Multiply/2
  Constant1/1 -> Subtract1/2
  Matrix Multiply2/1 -> Add1/1
  Matrix Multiply3/1 -> Add1/2
  tilt %1/1 -> Subtract1/1, Matrix Multiply2/2
  Subtract1/1 -> Matrix Multiply3/1
  Tilted Past Fit/1(Ct/Ct0 Tilted Past Fit) -> Matrix Multiply2/1
  Subsystem/1(Ct/Ct0 Non-tilt Past Fit) -> Matrix Multiply3/2
  Constant/1 -> Switch/1
  Uniform Random Number/1 -> Switch/3
  Switch/1 -> Add/3

== system dynamics/Quad Tiltrotor Dynamics/Airframe/Motor Forces and Torques/Multirotor Subsystem/Rotor Subsystem/Tilted Ct Estimator/Ct//C0 State Switcher/If Action Subsystem ==
  In1 : Inport
  Action Port : ActionPort  ActionPortLabel=if(u1 >= -2 & u1 <= 0)
  Out1 : Outport
  wires:
  In1/1 -> Out1/1

== system dynamics/Quad Tiltrotor Dynamics/Airframe/Motor Forces and Torques/Multirotor Subsystem/Rotor Subsystem/Tilted Ct Estimator/Ct//C0 State Switcher/If Action Subsystem1 ==
  Inport : Inport
  Action Port : ActionPort  ActionPortLabel=elseif(u1 < -2)
  " " : Outport
  wires:
  Inport/1 -> " "/1

== system dynamics/Quad Tiltrotor Dynamics/Airframe/Motor Forces and Torques/Multirotor Subsystem/Rotor Subsystem/Tilted Ct Estimator/Ct//C0 State Switcher/If Action Subsystem2 ==
  "  " : Inport
  Action Port : ActionPort  ActionPortLabel=else
  Out1 : Outport
  wires:
  "  "/1 -> Out1/1

== system dynamics/Quad Tiltrotor Dynamics/Airframe/Motor Forces and Torques/Multirotor Subsystem/Rotor Subsystem/Tilted Ct Estimator/Weighted Average Ct//C0 Fit/Subsystem ==
  " Vz/Vh" : Inport
  Add2 : Sum
  Constant : Constant  Value=2.07884583669
  Constant3 : Constant  Value=1.7439783573836165
  Gain : Gain  Gain=1/2
  Multiply : Gain  Gain=-1
  Saturation : Saturate  UpperLimit=inf  LowerLimit=0.0001
  Sum : Sum  Inputs=|++
  ln : Math  Operator=log
  Ct/Ct0 Non-tilt Past Fit : Outport
  wires:
  ln/1 -> Gain/1
  Sum/1 -> Multiply/1
  " Vz/Vh"/1 -> Sum/1
  Add2/1 -> Ct/Ct0 Non-tilt Past Fit/1
  Saturation/1 -> ln/1
  Multiply/1 -> Saturation/1
  Constant3/1 -> Sum/2
  Gain/1 -> Add2/1
  Constant/1 -> Add2/2

== system dynamics/Quad Tiltrotor Dynamics/Airframe/Motor Forces and Torques/Multirotor Subsystem/Rotor Subsystem/Tilted Ct Estimator/Weighted Average Ct//C0 Fit/Tilted Past Fit ==
  Vz/Vh : Inport
  Add1 : Sum
  Constant : Constant  Value=1.814813688
  Constant3 : Constant  Value=1.23626605195
  Gain : Gain  Gain=1/2
  Multiply : Gain  Gain=-1
  Saturation : Saturate  UpperLimit=inf  LowerLimit=0.001
  Sum : Sum  Inputs=|++
  ln : Math  Operator=log
  Ct/Ct0 Tilted Past Fit : Outport
  wires:
  Gain/1 -> Add1/1
  Saturation/1 -> ln/1
  Constant3/1 -> Sum/2
  Vz/Vh/1 -> Sum/1
  ln/1 -> Gain/1
  Multiply/1 -> Saturation/1
  Constant/1 -> Add1/2
  Add1/1 -> Ct/Ct0 Tilted Past Fit/1
  Sum/1 -> Multiply/1

== matlab function dynamics/Quad Tiltrotor Dynamics/Airframe/Motor Forces and Torques/Multirotor Subsystem/Rotor Subsystem/Induced Vel Convergence Checker ==
  data: rpmToCalc output; newVh output; Converged output; Vh input; convergence_threshold parameter; lastVh input
function [rpmToCalc, newVh, Converged] = CalculateInducedVelocity(Vh, convergence_threshold, lastVh)

    % Initialize variables
    persistent rpm_index rpm_values Vh_values exportedCoefficients;

    if isempty(rpm_index)
        rpm_index = 1;
        rpm_values = 1:1000:10001;
        Vh_values = zeros(size(rpm_values));
        exportedCoefficients = false;
    end

    if rpm_index > 11
        rpmToCalc = 1;
        newVh = 0.1;
        Converged = 1;
        return;
    end

    % Calculate the difference between the current and last induced velocity
    difference = abs(Vh - lastVh);
    rpmToCalc = rpm_values(rpm_index);

    if difference < convergence_threshold
        % Convergence achieved
        Converged = 1;
        newVh = Vh; % Update to the current induced velocity
        Vh_values(rpm_index) = Vh;
        
        if rpm_index >= length(rpm_values) && exportedCoefficients == false
            coefficients = fitVhToRPM(rpm_values, Vh_values);
            assignin('base', 'coefficients', coefficients);
            assignin('base', 'rpm_values', rpm_values);
            assignin('base', 'Vh_values', Vh_values);
            exportedCoefficients = true;
            return;
        else
            if rpm_index ~= 11
                rpmToCalc = rpm_values(rpm_index+1);
            end
        end

        % Move to the next RPM value
        if rpm_index < 11
            rpm_index = rpm_index + 1;
        end
    else
        % Convergence not achieved
        Converged = 0;
        newVh = Vh; % Update to the new induced velocity
    end
end

function coefficients = fitVhToRPM(rpm_values, Vh_values)
    % Fit a polynomial (or any other function) to the RPM and Vh values
    p = polyfit(rpm_values, Vh_values, 2);
    coefficients = p;
end
